simulink model "two_tanks_model_cascade_SIMC_ffwd_R2018"  (R2018a)
settings: Solver=VariableStepAuto  StartTime=0.0  StopTime=2400  FixedStep=0.1  RelTol=1e-3
model workspace (MATLAB code in the model file):
  | A1 = 1;
  | a1 = 0.1*0.1;
  | A2 = A1;
  | a2 = a1;
  | h10 = 1;
  | h20=1;
values from neighbouring files (symbols this model uses):
  Fv1 = K1    (= 14.5)    [two_tanks_cascade_ffwd.m]
  Fv2 = K1/K    (= 0.246878547106)    [two_tanks_cascade_ffwd.m]
  kc2 = 1    [two_tanks_cascade.m]    (also in two_tanks_cascade_ffwd.m)
  taui2 = t2    (= 59)    [two_tanks_cascade.m]    (also in two_tanks_cascade_ffwd.m)
settings Model: EnablePacing=on  PacingRate=35  Creator=kjartan  LastModifiedBy=kjartan
settings SFSimCC: SimUseLocalCustomCode=on
settings RTWCC: RTWUseLocalCustomCode=on

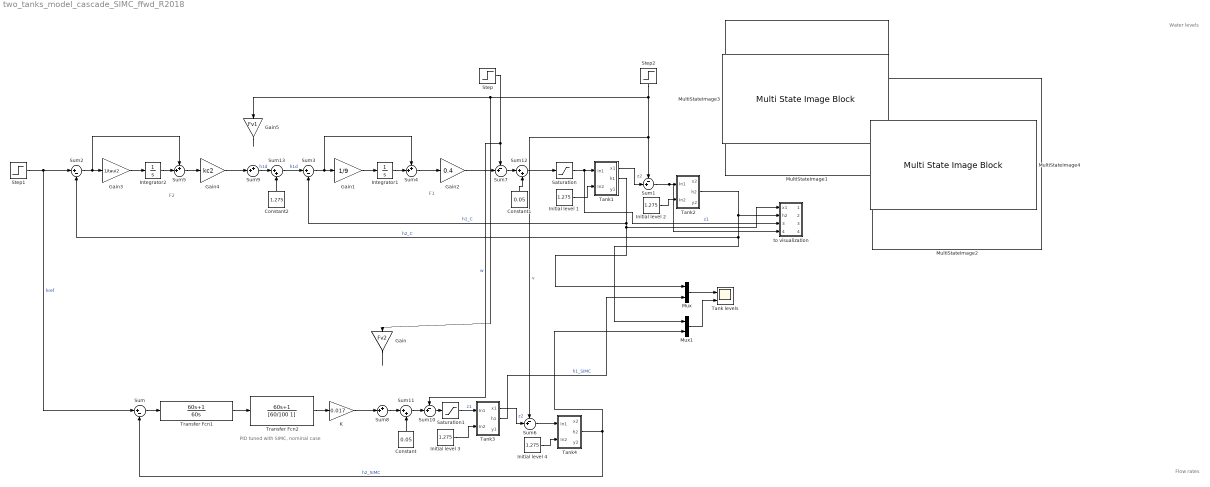
== system two_tanks_model_cascade_SIMC_ffwd_R2018 ==
  note: F2
  note: F1
  note: PID tuned with SIMC, nominal case
  note: Water levels
  note: Flow rates
  Constant : Constant  Value=0.05
  Constant1 : Constant  Value=0.05
  Constant2 : Constant  Value=1.275
  Gain : Gain  Gain=Fv2
  Gain1 : Gain  Gain=1/9
  Gain2 : Gain  Gain=0.4
  Gain3 : Gain  Gain=1/taui2
  Gain4 : Gain  Gain=kc2
  Gain5 : Gain  Gain=Fv1
  Initial level {1..4} (4 alike) : Constant  Value=1.275
  Integrator1 : Integrator
  Integrator2 : Integrator
  K : Gain  Gain=0.017
  MultiStateImage1 : MultiStateImageBlock  WebBlockId=219
  MultiStateImage2 : MultiStateImageBlock  WebBlockId=220
  MultiStateImage3 : MultiStateImageBlock  ScaleMode=Fill  WebBlockId=221
  MultiStateImage4 : MultiStateImageBlock  ScaleMode=Fill  WebBlockId=222
  Mux : Mux  Inputs=2
  Mux1 : Mux  Inputs=2
  Saturation : Saturate  LowerLimit=0
  Saturation1 : Saturate  LowerLimit=0
  Step : Step  Time=800  After=0.015  SampleTime=0
  Step1 : Step  Time=120  Before=1.275  After=2  SampleTime=0
  Step2 : Step  Time=1600  After=0.01  SampleTime=0
  Sum : Sum  Inputs=|+-
  Sum{1,6..7,10} (4 alike) : Sum  Inputs=-+|
  Sum11 : Sum  Inputs=|++
  Sum12 : Sum  Inputs=|++
  Sum13 : Sum  Inputs=|++
  Sum2 : Sum  Inputs=|+-
  Sum3 : Sum  Inputs=|+-
  Sum{4..5,8..9} (4 alike) : Sum  Inputs=++|
  Tank levels : Scope  NumInputPorts=2
  Tank1 : Subsystem
  Tank2 : Subsystem
  Tank3 : Subsystem
  Tank4 : Subsystem
  Transfer Fcn1 : TransferFcn  Numerator=[60, 1]  Denominator=[60 0]
  Transfer Fcn2 : TransferFcn  Numerator=[60, 1]  Denominator=[60/100 1]
  to visualization : Subsystem
  wires:
  Tank1/1(x1) -> Sum1/2  "z2"
  Tank1/2(h1) -> to visualization/1(x1), Mux/1, Sum3/2  "h1_C"
  Sum1/1 -> to visualization/4(In4), Tank2/1(In1)
  Saturation/1 -> to visualization/3(In3), Tank1/1(In1)  "z1"
  Initial level 2/1 -> Tank2/2(In2)
  Initial level 1/1 -> Tank1/2(In2)
  Step2/1 -> Gain/1, Gain5/1, Sum6/1, Sum1/1  "v"
  Gain1/1 -> Integrator1/1
  Integrator1/1 -> Sum4/2
  Sum3/1 -> Sum4/1, Gain1/1
  Sum4/1 -> Gain2/1
  Gain2/1 -> Sum7/2
  Gain3/1 -> Integrator2/1
  Tank2/2(h2) -> Mux1/1, Sum2/2, to visualization/2(h2)  "h2_C"
  Gain4/1 -> Sum9/2
  Sum2/1 -> Sum5/1, Gain3/1
  Sum5/1 -> Gain4/1
  Integrator2/1 -> Sum5/2
  Transfer Fcn2/1 -> K/1
  Initial level 3/1 -> Tank3/2(In2)
  Saturation1/1 -> Tank3/1(In1)  "z1"
  Tank3/2(h1) -> Mux/2  "h1_SIMC"
  K/1 -> Sum8/2
  Initial level 4/1 -> Tank4/2(In2)
  Step1/1 -> Sum/1, Sum2/1  "href"
  Sum/1 -> Transfer Fcn1/1
  Sum6/1 -> Tank4/1(In1)
  Tank3/1(x1) -> Sum6/2  "z2"
  Transfer Fcn1/1 -> Transfer Fcn2/1
  Tank4/2(h2) -> Sum/2, Mux1/2  "h2_SIMC"
  Mux/1 -> Tank levels/1
  Mux1/1 -> Tank levels/2
  Step/1 -> Sum10/1, Sum7/1  "w"
  Sum8/1 -> Sum11/1
  Sum7/1 -> Sum12/1
  Sum10/1 -> Saturation1/1
  Gain/1 -> ?
  Sum9/1 -> Sum13/1  "h1d"
  Gain5/1 -> ?
  Sum11/1 -> Sum10/2
  Constant/1 -> Sum11/2
  Sum12/1 -> Saturation/1
  Constant1/1 -> Sum12/2
  Sum13/1 -> Sum3/1  "h1d"
  Constant2/1 -> Sum13/2

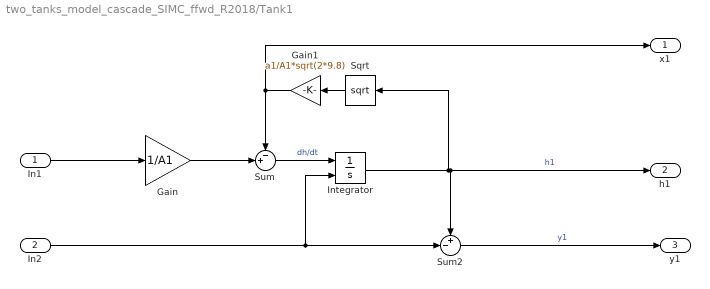
== system two_tanks_model_cascade_SIMC_ffwd_R2018/Tank1 ==
  In1 : Inport
  In2 : Inport  Port=2
  Gain : Gain  Gain=1/A1
  Gain1 : Gain  Gain=a1/A1*sqrt(2*9.8)
  Integrator : Integrator  InitialConditionSource=external  InitialCondition=h10  LimitOutput=on  LowerSaturationLimit=0
  Sqrt : Sqrt  SaturateOnIntegerOverflow=on
  Sum : Sum  Inputs=-+|
  Sum2 : Sum  Inputs=+-|
  x1 : Outport  VectorParamsAs1DForOutWhenUnconnected=off
  h1 : Outport  Port=2  VectorParamsAs1DForOutWhenUnconnected=off
  y1 : Outport  Port=3  VectorParamsAs1DForOutWhenUnconnected=off
  wires:
  Gain1/1 -> x1/1, Sum/1
  Gain/1 -> Sum/2
  Sum/1 -> Integrator/1  "dh/dt"
  In1/1 -> Gain/1
  Sum2/1 -> y1/1  "y1"
  Sqrt/1 -> Gain1/1
  Integrator/1 -> Sqrt/1, h1/1, Sum2/1  "h1"
  In2/1 -> Sum2/2, Integrator/2

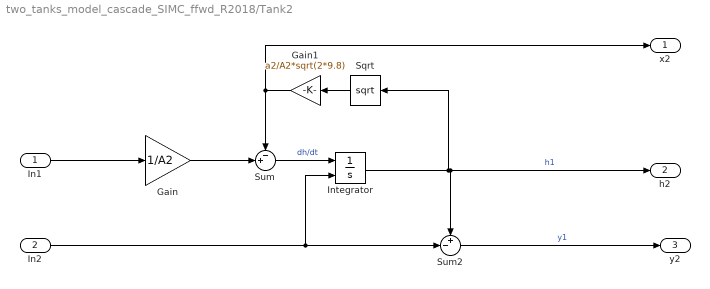
== system two_tanks_model_cascade_SIMC_ffwd_R2018/Tank2 ==
  In1 : Inport
  In2 : Inport  Port=2
  Gain : Gain  Gain=1/A2
  Gain1 : Gain  Gain=a2/A2*sqrt(2*9.8)
  Integrator : Integrator  InitialConditionSource=external  InitialCondition=h10  LimitOutput=on  LowerSaturationLimit=0
  Sqrt : Sqrt  SaturateOnIntegerOverflow=on
  Sum : Sum  Inputs=-+|
  Sum2 : Sum  Inputs=+-|
  x2 : Outport  VectorParamsAs1DForOutWhenUnconnected=off
  h2 : Outport  Port=2  VectorParamsAs1DForOutWhenUnconnected=off
  y2 : Outport  Port=3  VectorParamsAs1DForOutWhenUnconnected=off
  wires:
  Gain1/1 -> x2/1, Sum/1
  Gain/1 -> Sum/2
  Sum/1 -> Integrator/1  "dh/dt"
  In1/1 -> Gain/1
  Sum2/1 -> y2/1  "y1"
  Sqrt/1 -> Gain1/1
  Integrator/1 -> Sqrt/1, h2/1, Sum2/1  "h1"
  In2/1 -> Sum2/2, Integrator/2

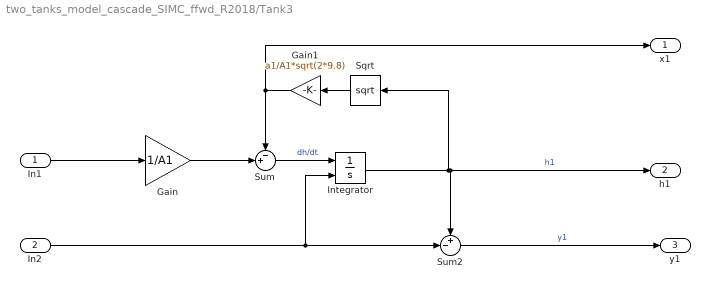
== system two_tanks_model_cascade_SIMC_ffwd_R2018/Tank3 ==
  In1 : Inport
  In2 : Inport  Port=2
  Gain : Gain  Gain=1/A1
  Gain1 : Gain  Gain=a1/A1*sqrt(2*9.8)
  Integrator : Integrator  InitialConditionSource=external  InitialCondition=h10  LimitOutput=on  LowerSaturationLimit=0
  Sqrt : Sqrt  SaturateOnIntegerOverflow=on
  Sum : Sum  Inputs=-+|
  Sum2 : Sum  Inputs=+-|
  x1 : Outport  VectorParamsAs1DForOutWhenUnconnected=off
  h1 : Outport  Port=2  VectorParamsAs1DForOutWhenUnconnected=off
  y1 : Outport  Port=3  VectorParamsAs1DForOutWhenUnconnected=off
  wires:
  Gain1/1 -> x1/1, Sum/1
  Gain/1 -> Sum/2
  Sum/1 -> Integrator/1  "dh/dt"
  In1/1 -> Gain/1
  Sum2/1 -> y1/1  "y1"
  Sqrt/1 -> Gain1/1
  Integrator/1 -> Sqrt/1, h1/1, Sum2/1  "h1"
  In2/1 -> Sum2/2, Integrator/2

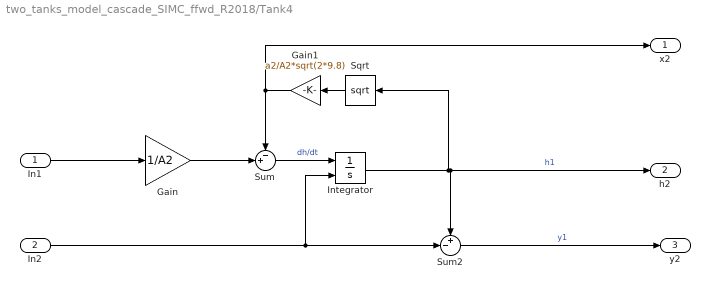
== system two_tanks_model_cascade_SIMC_ffwd_R2018/Tank4 ==
  In1 : Inport
  In2 : Inport  Port=2
  Gain : Gain  Gain=1/A2
  Gain1 : Gain  Gain=a2/A2*sqrt(2*9.8)
  Integrator : Integrator  InitialConditionSource=external  InitialCondition=h10  LimitOutput=on  LowerSaturationLimit=0
  Sqrt : Sqrt  SaturateOnIntegerOverflow=on
  Sum : Sum  Inputs=-+|
  Sum2 : Sum  Inputs=+-|
  x2 : Outport  VectorParamsAs1DForOutWhenUnconnected=off
  h2 : Outport  Port=2  VectorParamsAs1DForOutWhenUnconnected=off
  y2 : Outport  Port=3  VectorParamsAs1DForOutWhenUnconnected=off
  wires:
  Gain1/1 -> x2/1, Sum/1
  Gain/1 -> Sum/2
  Sum/1 -> Integrator/1  "dh/dt"
  In1/1 -> Gain/1
  Sum2/1 -> y2/1  "y1"
  Integrator/1 -> Sqrt/1, h2/1, Sum2/1  "h1"
  In2/1 -> Sum2/2, Integrator/2
  Sqrt/1 -> Gain1/1

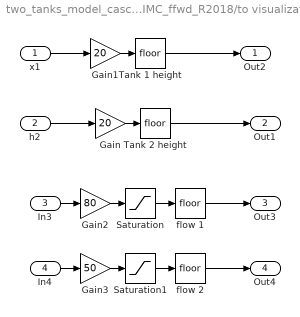
== system two_tanks_model_cascade_SIMC_ffwd_R2018/to visualization ==
  x1 : Inport
  h2 : Inport  Port=2
  In3 : Inport  Port=3
  In4 : Inport  Port=4
  Gain : Gain  Gain=20
  Gain1 : Gain  Gain=20
  Gain2 : Gain  Gain=80
  Gain3 : Gain  Gain=50
  Saturation : Saturate  UpperLimit=10  LowerLimit=0
  Saturation1 : Saturate  UpperLimit=5  LowerLimit=0
  Tank 1 height : Rounding
  Tank 2 height : Rounding
  flow 1 : Rounding
  flow 2 : Rounding
  Out2 : Outport  VectorParamsAs1DForOutWhenUnconnected=off
  Out1 : Outport  Port=2  VectorParamsAs1DForOutWhenUnconnected=off
  Out3 : Outport  Port=3  VectorParamsAs1DForOutWhenUnconnected=off
  Out4 : Outport  Port=4  VectorParamsAs1DForOutWhenUnconnected=off
  wires:
  Tank 2 height/1 -> Out1/1
  Gain/1 -> Tank 2 height/1
  h2/1 -> Gain/1
  Tank 1 height/1 -> Out2/1
  Gain1/1 -> Tank 1 height/1
  x1/1 -> Gain1/1
  flow 1/1 -> Out3/1
  Gain2/1 -> Saturation/1
  In3/1 -> Gain2/1
  flow 2/1 -> Out4/1
  In4/1 -> Gain3/1
  Gain3/1 -> Saturation1/1
  Saturation/1 -> flow 1/1
  Saturation1/1 -> flow 2/1
